simulink library "HyEQ_Library_R2012a"  (R2017a)
settings: Solver=ode45  StartTime=0.0  StopTime=T  MaxStep=MaxStep  RelTol=RelTol  EnableMultiTasking=on
undefined symbols (not defined in the file): C, D, f, g, J, maxU, maxX, minU, rule, T, Tnmax, Tnmin, x0, x0ADC, x0NET
libraries: simulink x24
(part 1 of 3)
settings Model: Creator=pablonanez  LastModifiedBy=pablonanez
settings DataIOCC: LimitDataPoints=on  SaveFormat=Array  SignalLoggingSaveFormat=ModelDataLogs
settings OptimizationCC: ExpressionDepthLimit=2147483647  LifeSpan=inf
settings DebuggingCC: UnderspecifiedInitializationDetection=Classic  MergeDetectMultiDrivingBlocksExec=none  SolverPrmCheckMsg=warning  FcnCallInpInsideContextMsg=warning  StateNameClashWarn=warning  SFUnexpectedBacktrackingDiag=warning  SFNoUnconditionalDefaultTransitionDiag=warning  SFExecutionAtInitializationDiag=none
settings HardwareCC: ProdBitPerPointer=32  ProdBitPerSizeT=32  ProdBitPerPtrDiffT=32  ProdLargestAtomicFloat=None  ProdIntDivRoundTo=Undefined  ProdEndianess=Unspecified  ProdWordSize=32  ProdHWDeviceType=32-bit Generic
settings ModelReferenceCC: PropagateSignalLabelsOutOfModel=off
settings GRTTargetCC: TargetLangStandard=C89/C90 (ANSI)  GeneratePreprocessorConditionals=Disable all  CombineOutputUpdateFcns=off  GRTInterface=on
settings ConfigComp: CovMetricSettings=dw  CovHtmlReporting=on  CovSaveCumulativeToWorkspaceVar=on  CovSaveSingleToWorkspaceVar=on  CovExternalEMLEnable=off

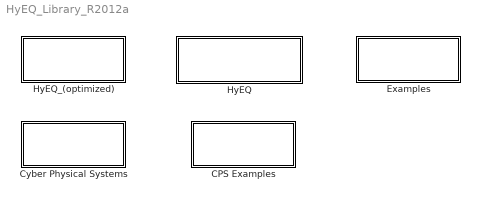
== system HyEQ_Library_R2012a ==
  CPS Examples : Subsystem  LoadFcn=set_param(gcb,'LinkStatus','none')
      settings: CopyFcn=set_param(gcb,'LinkStatus','none')
      mask Display: disp('CPS\n Examples')
  Cyber Physical Systems : Subsystem  LoadFcn=set_param(gcb,'LinkStatus','none')
      settings: CopyFcn=set_param(gcb,'LinkStatus','none')
      mask Display: disp('CPS')
  Examples : Subsystem  LoadFcn=set_param(gcb,'LinkStatus','none')
      settings: CopyFcn=set_param(gcb,'LinkStatus','none')
      mask Display: disp('HyEQ\n Examples')
  HyEQ : Subsystem  LoadFcn=set_param(gcb,'LinkStatus','none')
      settings: CopyFcn=set_param(gcb,'LinkStatus','none')
      mask Display:
      | color('white')
      | 
      | disp('HyEQ \n (No C compiler required)')
  HyEQ_(optimized) : Subsystem  LoadFcn=set_param(gcb,'LinkStatus','none')
      settings: CopyFcn=set_param(gcb,'LinkStatus','none')
      mask Display: disp('HyEQ \n (optimized)')

== system HyEQ_Library_R2012a/CPS Examples ==
  ADC Example 1 : Subsystem  LoadFcn=set_param(gcb,'LinkStatus','none')  mask(Help for the bouncing ball example){}
      mask help: Example: Bouncing ball
      settings: CopyFcn=set_param(gcb,'LinkStatus','none')  OpenFcn=open_system('ADC_example1','force')
      mask Display: disp('ADC example 1')
  ADC Example 2 : Subsystem  LoadFcn=set_param(gcb,'LinkStatus','none')  mask(Help for the bouncing ball example){}
      mask help: Example: Bouncing ball
      settings: CopyFcn=set_param(gcb,'LinkStatus','none')  OpenFcn=open_system('ADC_example2','force')
      mask Display: disp('ADC example 2')
  Continuous Plant : Subsystem  LoadFcn=set_param(gcb,'LinkStatus','none')  mask(Help for the bouncing ball example){}
      mask help: Example: Bouncing ball
      settings: CopyFcn=set_param(gcb,'LinkStatus','none')  OpenFcn=open_system('ContinuousPlant_example','force')
      mask Display: disp('Continuous plant example')
  Finite State Machine Example : Subsystem  LoadFcn=set_param(gcb,'LinkStatus','none')  mask(Help for the bouncing ball example){}
      mask help: Example: Bouncing ball
      settings: CopyFcn=set_param(gcb,'LinkStatus','none')  OpenFcn=open_system('FSM_example','force')
      mask Display: disp('FSM example')
  Networks : Subsystem  LoadFcn=set_param(gcb,'LinkStatus','none')  mask(Help for the bouncing ball example){}
      mask help: Example: Bouncing ball
      settings: CopyFcn=set_param(gcb,'LinkStatus','none')  OpenFcn=open_system('Network_example','force')
      mask Display: disp('Network example')
  Zero Order Hold Example : Subsystem  LoadFcn=set_param(gcb,'LinkStatus','none')  mask(Help for the bouncing ball example){}
      mask help: Example: Bouncing ball
      settings: CopyFcn=set_param(gcb,'LinkStatus','none')  OpenFcn=open_system('ZOH_example','force')
      mask Display: disp('ZOH example')

== system HyEQ_Library_R2012a/Cyber Physical Systems ==
  ADC : Subsystem  LoadFcn=set_param(gcb,'LinkStatus','none')
      settings: CopyFcn=|
      | set_param(gcb,'LinkStatus','none'),
      | set_param(gcs, 'MaxStep', 'MaxStep', 'RelTol', 'RelTol','Stop time', 'T')
      mask Display:
      | image(imread('ADC.jpg'))
      | %plot([5 20 20 5 5],[5 5 20 20 5])
      | %text(8,13,'HyEq_mdl')
      | port_label('output', 1, 'x')
      | port_label('output', 2, 't')
      | port_label('output', 3, 'j')
      | port_label('output', 4, 'x-(int)')
      | port_label('input', 1, 'u')
  FSM : Subsystem  LoadFcn=set_param(gcb,'LinkStatus','none')
      settings: CopyFcn=|
      | set_param(gcb,'LinkStatus','none'),
      | set_param(gcs, 'MaxStep', 'MaxStep', 'RelTol', 'RelTol','Stop time', 'T')
      mask Display:
      | image(imread('FSM.jpg'))
      | %plot([5 20 20 5 5],[5 5 20 20 5])
      | %text(8,13,'HyEq_mdl')
      | port_label('output', 1, 'x')
      | port_label('output', 2, 't')
      | port_label('output', 3, 'j')
      | port_label('output', 4, 'x-(int)')
      | port_label('input', 1, 'u')
  HSu : Subsystem  LoadFcn=set_param(gcb,'LinkStatus','none')
      settings: CopyFcn=|
      | set_param(gcb,'LinkStatus','none'),
      | set_param(gcs, 'MaxStep', 'MaxStep', 'RelTol', 'RelTol','Stop time', 'T')
      mask Display:
      | image(imread('Cplant.jpg'))
      | %plot([5 20 20 5 5],[5 5 20 20 5])
      | %text(8,13,'HyEq_mdl')
      | port_label('output', 1, 'x')
      | port_label('output', 2, 't')
      | port_label('output', 3, 'j')
      | port_label('output', 4, 'x-(int)')
      | port_label('input', 1, 'u')
  ZOH : Subsystem  LoadFcn=set_param(gcb,'LinkStatus','none')
      settings: CopyFcn=|
      | set_param(gcb,'LinkStatus','none'),
      | set_param(gcs, 'MaxStep', 'MaxStep', 'RelTol', 'RelTol','Stop time', 'T')
      mask Display:
      | image(imread('ZOH.jpg'))
      | %plot([5 20 20 5 5],[5 5 20 20 5])
      | %text(8,13,'HyEq_mdl')
      | port_label('output', 1, 'x')
      | port_label('output', 2, 't')
      | port_label('output', 3, 'j')
      | port_label('output', 4, 'x-(int)')
      | port_label('input', 1, 'u')
  network : Subsystem  LoadFcn=set_param(gcb,'LinkStatus','none')
      settings: CopyFcn=|
      | set_param(gcb,'LinkStatus','none'),
      | set_param(gcs, 'MaxStep', 'MaxStep', 'RelTol', 'RelTol','Stop time', 'T')
      mask Display:
      | image(imread('net.jpg'))
      | %plot([5 20 20 5 5],[5 5 20 20 5])
      | %text(8,13,'HyEq_mdl')
      | port_label('output', 1, 'x')
      | port_label('output', 2, 't')
      | port_label('output', 3, 'j')
      | port_label('output', 4, 'x-(int)')
      | port_label('input', 1, 'u')

== system HyEQ_Library_R2012a/Examples ==
  Ex 1.2a Bouncing ball example : Subsystem  LoadFcn=set_param(gcb,'LinkStatus','none')  mask(Help for the bouncing ball example){}
      mask help: Example: Bouncing ball
      settings: CopyFcn=set_param(gcb,'LinkStatus','none')  OpenFcn=open_system('Example_1_2a','force')
      mask Display: disp('Ex 1.2a Bouncing ball \n (external functions)')
  Ex 1.3 Bouncing ball with input : Subsystem  LoadFcn=set_param(gcb,'LinkStatus','none')  mask(Help for the bouncing ball example){}
      mask help: Example: Bouncing ball
      settings: CopyFcn=set_param(gcb,'LinkStatus','none')  OpenFcn=open_system('Example1_3','force')
      mask Display: disp('Ex 1.3 Bouncing ball \n (with input)')
  Ex 1.4 Bouncing ball with operator blocks : Subsystem  LoadFcn=set_param(gcb,'LinkStatus','none')  mask(Help for the bouncing ball example){}
      mask help: Example: Bouncing ball
      settings: CopyFcn=set_param(gcb,'LinkStatus','none')  OpenFcn=open_system('Example1_4','force')
      mask Display: disp('Ex 1.4 Bouncing ball \n (operator blocks)')
  Ex 1.5 Vehicle on Path with Boundaries : Subsystem  LoadFcn=set_param(gcb,'LinkStatus','none')  mask(Help for the bouncing ball example){}
      mask help: Example: Bouncing ball
      settings: CopyFcn=set_param(gcb,'LinkStatus','none')  OpenFcn=open_system('Example1_5','force')
      mask Display: disp('Ex 1.5 Vehicle on Path')
  Ex 1.6 Bouncing Ball and Plataform : Subsystem  LoadFcn=set_param(gcb,'LinkStatus','none')  mask(Help for the bouncing ball example){}
      mask help: Example: Bouncing ball
      settings: CopyFcn=set_param(gcb,'LinkStatus','none')  OpenFcn=open_system('Example1_6','force')
      mask Display: disp('Ex 1.6 Bouncing Ball \n and Moving Platform')
  Ex 1.7 Synchronization of Fireflies : Subsystem  LoadFcn=set_param(gcb,'LinkStatus','none')  mask(Help for the bouncing ball example){}
      mask help: Example: Bouncing ball
      settings: CopyFcn=set_param(gcb,'LinkStatus','none')  OpenFcn=open_system('Example1_7','force')
      mask Display: disp('Ex 1.7 Fireflies')
  Ex 1.8 a Simple Example : Subsystem  LoadFcn=set_param(gcb,'LinkStatus','none')  mask(Help for a simple mathematical example){}
      mask help: Example: a simple mathematical example
      settings: CopyFcn=set_param(gcb,'LinkStatus','none')  OpenFcn=open_system('Ex_1_8_Subblocks','force')
      mask Display: disp('Ex 1.8 a Simple \n Example')

== system HyEQ_Library_R2012a/HyEQ ==
  HS : Subsystem  LoadFcn=set_param(gcb,'LinkStatus','none')
      settings: CopyFcn=|
      | set_param(gcb,'LinkStatus','none'),
      | set_param(gcs, 'MaxStep', 'MaxStep', 'RelTol', 'RelTol')
      mask Display:
      | image(imread('Hcalneg.jpg'))
      | %plot([5 20 20 5 5],[5 5 20 20 5])
      | %text(8,13,'HyEq_mdl')
      | color('white')
      | port_label('output', 1, 'x')
      | port_label('output', 2, 't')
      | port_label('output', 3, 'j')
  Initialize variables : Subsystem  Priority=-10  mask(Initialization file load){}
      mask help: Select the initialization script
      settings: OpenFcn=|
      | try
      |      clearvars -except inifile pathfile_in pathfile_pos posfile
      |      cd(pathfile_in);
      |      eval(inifile);
      | catch
      |      [inifile,pathfile_in] = getInitializationfile;
      |      cd(pathfile_in);
      |      inifile = strrep(inifile,'.m','');
      |      eval(inifile);
      | end
      mask Display: disp('Double Click\n to Initialize')
  More info : Subsystem  mask(Help for HyEQ blocks){}
      mask help: How to use the HyEQ simulink blocks
      settings: OpenFcn=|
      | try
      |      open_system('HyEQ_No_C_Compiler','force')       catch
      | end
      mask Display: disp('Help')
  Plot Solutions : Subsystem  mask(Postprocesing file load){}
      mask help: Select the postprocesing script
      settings: OpenFcn=|
      | try
      |      cd(pathfile_pos);
      |      eval(posfile);
      | catch
      |      [posfile,pathfile_pos] = getInitializationfile;
      |      cd(pathfile_pos);
      |      posfile = strrep(posfile,'.m','');
      |      eval(posfile);
      | end
      mask Display: disp('Double Click to\n Plot Solutions')

== system HyEQ_Library_R2012a/HyEQ_(optimized) ==
  HS : Subsystem  LoadFcn=set_param(gcb,'LinkStatus','none')
      settings: CopyFcn=|
      | set_param(gcb,'LinkStatus','none'),
      | set_param(gcs, 'MaxStep', 'MaxStep', 'RelTol', 'RelTol','Stop time', 'T')
      mask Display:
      | image(imread('Hcal.jpg'))
      | %plot([5 20 20 5 5],[5 5 20 20 5])
      | %text(8,13,'HyEq_mdl')
      | port_label('output', 1, 'x')
      | port_label('output', 2, 't')
      | port_label('output', 3, 'j')
  HSu : Subsystem  LoadFcn=set_param(gcb,'LinkStatus','none')
      settings: CopyFcn=|
      | set_param(gcb,'LinkStatus','none'),
      | set_param(gcs, 'MaxStep', 'MaxStep', 'RelTol', 'RelTol','Stop time', 'T')
      mask Display:
      | image(imread('Hcal.jpg'))
      | %plot([5 20 20 5 5],[5 5 20 20 5])
      | %text(8,13,'HyEq_mdl')
      | port_label('output', 1, 'x')
      | port_label('output', 2, 't')
      | port_label('output', 3, 'j')
      | port_label('output', 4, 'x-(int)')
      | port_label('input', 1, 'u')
  Initialize variables : Subsystem  Priority=-10  mask(Initialization file load){}
      mask help: Select the initialization script
      settings: OpenFcn=|
      | try
      |      clearvars -except inifile pathfile_in pathfile_pos posfile
      |      cd(pathfile_in);
      |      eval(inifile);
      | catch
      |      [inifile,pathfile_in] = getInitializationfile;
      |      cd(pathfile_in);
      |      inifile = strrep(inifile,'.m','');
      |      eval(inifile);
      | end
      mask Display: disp('Double Click\n to Initialize')
  More info : Subsystem  mask(Help for HyEQ blocks){}
      mask help: How to use the HyEQ simulink blocks
      settings: OpenFcn=|
      | try
      |      open_system('HyEQ_Optimized','force')
      | catch
      | end
      mask Display: disp('Help')
  Plot Solutions : Subsystem  mask(Postprocesing file load){}
      mask help: Select the postprocesing script
      settings: OpenFcn=|
      | try
      |      cd(pathfile_pos);
      |      eval(posfile);
      | catch
      |      [posfile,pathfile_pos] = getInitializationfile;
      |      cd(pathfile_pos);
      |      posfile = strrep(posfile,'.m','');
      |      eval(posfile);
      | end
      mask Display: disp('Double Click to\n Plot Solutions')

== system HyEQ_Library_R2012a/CPS Examples/ADC Example 1 ==
  Gain : Gain

== system HyEQ_Library_R2012a/CPS Examples/ADC Example 2 ==
  Gain : Gain

== system HyEQ_Library_R2012a/CPS Examples/Continuous Plant ==
  Gain : Gain

== system HyEQ_Library_R2012a/CPS Examples/Finite State Machine Example ==
  Gain : Gain

== system HyEQ_Library_R2012a/CPS Examples/Networks ==
  Gain : Gain

== system HyEQ_Library_R2012a/CPS Examples/Zero Order Hold Example ==
  Gain : Gain

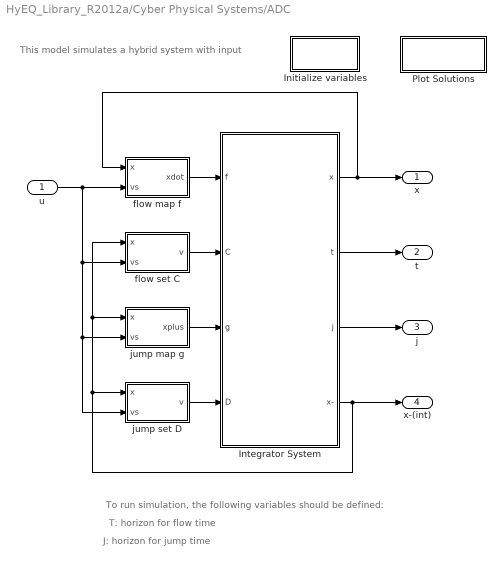
== system HyEQ_Library_R2012a/Cyber Physical Systems/ADC ==
  note: This model simulates a hybrid system with input
  note: To run simulation, the following variables should be defined:
  note: T: horizon for flow time
  note: J: horizon for jump time
  u : Inport
  Initialize variables : Subsystem  Priority=-10
      settings: OpenFcn=|
      | try
      |      clearvars -except inifile pathfile_in pathfile_pos posfile
      |      cd(pathfile_in);
      |      eval(inifile);
      | catch
      |      [inifile,pathfile_in] = getInitializationfile;
      |      cd(pathfile_in);
      |      inifile = strrep(inifile,'.m','');
      |      eval(inifile);
      | end
      mask Display: disp('Double Click\n to Initialize')
  Integrator System : Subsystem  Priority=2  mask(Hybrid Integrator){T=T, J=J, x0=x0ADC}
      mask prompts: T "Flow Horizon"; J "Jump Horizon"; x0 "Initial Condition"
      mask help:
      | This block integrates the state of the hybrid system defined by the flow map f (first input), the flow set C (second input), the jump map g (third input) and the jump set D (fourth input).
      | Starting from the initial condition x0 (last mask parameter), the system's state x evolves continuously within the set C, according to f(x,u), but is also subject to jumps within D, according to g(x,u).
      | The block also stops the simulation when the time t is greater than the flow horizon T (first mask parameter), or when the number of jumps j is greater than the jump horizon J (second mask parameter).
      | The outputs of the blocks are respectively x(t), t, j, x(t-).
      mask Help:
      | This block integrates the state of the hybrid system defined by the flow map f (first input), the flow set C (second input), the jump map g (third input) and the jump set D (fourth input).
      | <br>
      | Starting from the initial condition x0 (last mask parameter), the system's state x evolves continuously within the set C, according to f(x,u), but is also subject to jumps within D, according to g(x,u).
      | <br>
      | The block also stops the simulation when the time t is greater than the flow horizon T (first mask parameter), or when the number of jumps j is greater than the jump horizon J (second mask parameter).
      | <br>
      | The outputs of the blocks are respectively x(t), t, j, x(t-).
      | <br>
      | You can right click on the block and "Look under mask" to see what's inside the block.
      | Finally, refer to the manual (HybridSimulator_vXX.pdf) for more detailed information on how this hybrid simulator works.
  Plot Solutions : Subsystem
      settings: OpenFcn=|
      | try
      |      cd(pathfile_pos);
      |      eval(posfile);
      | catch
      |      [posfile,pathfile_pos] = getInitializationfile;
      |      cd(pathfile_pos);
      |      posfile = strrep(posfile,'.m','');
      |      eval(posfile);
      | end
      mask Display: disp('Double Click to\n Plot Solutions')
  flow map f : MATLAB Function  TreatAsAtomicUnit=on
  flow set C : MATLAB Function  TreatAsAtomicUnit=on
  jump map g : MATLAB Function  Priority=2  TreatAsAtomicUnit=on
  jump set D : MATLAB Function  TreatAsAtomicUnit=on
  x : Outport
  t : Outport  Port=2
  j : Outport  Port=3
  x-(int) : Outport  Port=4
  wires:
  flow map f/1(xdot) -> Integrator System/1(f)
  Integrator System/4(x-) -> jump map g/1(x), flow set C/1(x), jump set D/1(x), x-(int)/1
  Integrator System/1(x) -> flow map f/1(x), x/1
  flow set C/1(v) -> Integrator System/2(C)
  Integrator System/2(t) -> t/1
  Integrator System/3(j) -> j/1
  u/1 -> flow map f/2(vs), flow set C/2(vs), jump map g/2(vs), jump set D/2(vs)
  jump set D/1(v) -> Integrator System/4(D)
  jump map g/1(xplus) -> Integrator System/3(g)

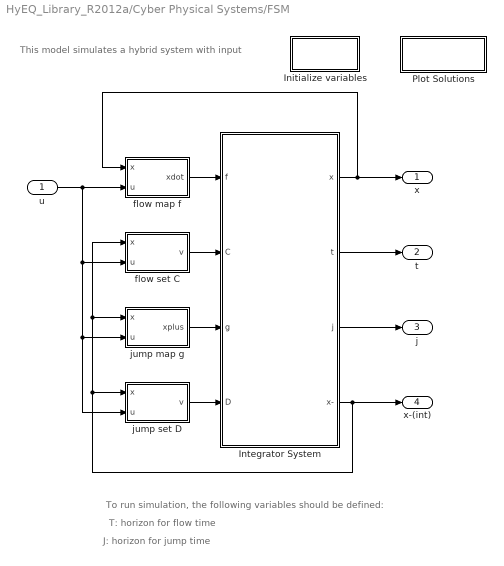
== system HyEQ_Library_R2012a/Cyber Physical Systems/FSM ==
  note: This model simulates a hybrid system with input
  note: To run simulation, the following variables should be defined:
  note: T: horizon for flow time
  note: J: horizon for jump time
  u : Inport
  Initialize variables : Subsystem  Priority=-10
      settings: OpenFcn=|
      | try
      |      clearvars -except inifile pathfile_in pathfile_pos posfile
      |      cd(pathfile_in);
      |      eval(inifile);
      | catch
      |      [inifile,pathfile_in] = getInitializationfile;
      |      cd(pathfile_in);
      |      inifile = strrep(inifile,'.m','');
      |      eval(inifile);
      | end
      mask Display: disp('Double Click\n to Initialize')
  Integrator System : Subsystem  Priority=2  mask(Hybrid Integrator){T=T, J=J, x0=x0}
      mask prompts: T "Flow Horizon"; J "Jump Horizon"; x0 "Initial Condition"
      mask help:
      | This block integrates the state of the hybrid system defined by the flow map f (first input), the flow set C (second input), the jump map g (third input) and the jump set D (fourth input).
      | Starting from the initial condition x0 (last mask parameter), the system's state x evolves continuously within the set C, according to f(x,u), but is also subject to jumps within D, according to g(x,u).
      | The block also stops the simulation when the time t is greater than the flow horizon T (first mask parameter), or when the number of jumps j is greater than the jump horizon J (second mask parameter).
      | The outputs of the blocks are respectively x(t), t, j, x(t-).
      mask Help:
      | This block integrates the state of the hybrid system defined by the flow map f (first input), the flow set C (second input), the jump map g (third input) and the jump set D (fourth input).
      | <br>
      | Starting from the initial condition x0 (last mask parameter), the system's state x evolves continuously within the set C, according to f(x,u), but is also subject to jumps within D, according to g(x,u).
      | <br>
      | The block also stops the simulation when the time t is greater than the flow horizon T (first mask parameter), or when the number of jumps j is greater than the jump horizon J (second mask parameter).
      | <br>
      | The outputs of the blocks are respectively x(t), t, j, x(t-).
      | <br>
      | You can right click on the block and "Look under mask" to see what's inside the block.
      | Finally, refer to the manual (HybridSimulator_vXX.pdf) for more detailed information on how this hybrid simulator works.
  Plot Solutions : Subsystem
      settings: OpenFcn=|
      | try
      |      cd(pathfile_pos);
      |      eval(posfile);
      | catch
      |      [posfile,pathfile_pos] = getInitializationfile;
      |      cd(pathfile_pos);
      |      posfile = strrep(posfile,'.m','');
      |      eval(posfile);
      | end
      mask Display: disp('Double Click to\n Plot Solutions')
  flow map f : MATLAB Function  TreatAsAtomicUnit=on
  flow set C : MATLAB Function  TreatAsAtomicUnit=on
  jump map g : MATLAB Function  Priority=2  TreatAsAtomicUnit=on
  jump set D : MATLAB Function  TreatAsAtomicUnit=on
  x : Outport
  t : Outport  Port=2
  j : Outport  Port=3
  x-(int) : Outport  Port=4
  wires:
  flow map f/1(xdot) -> Integrator System/1(f)
  Integrator System/4(x-) -> jump map g/1(x), flow set C/1(x), jump set D/1(x), x-(int)/1
  Integrator System/1(x) -> flow map f/1(x), x/1
  flow set C/1(v) -> Integrator System/2(C)
  Integrator System/2(t) -> t/1
  Integrator System/3(j) -> j/1
  u/1 -> flow map f/2(u), flow set C/2(u), jump map g/2(u), jump set D/2(u)
  jump set D/1(v) -> Integrator System/4(D)
  jump map g/1(xplus) -> Integrator System/3(g)

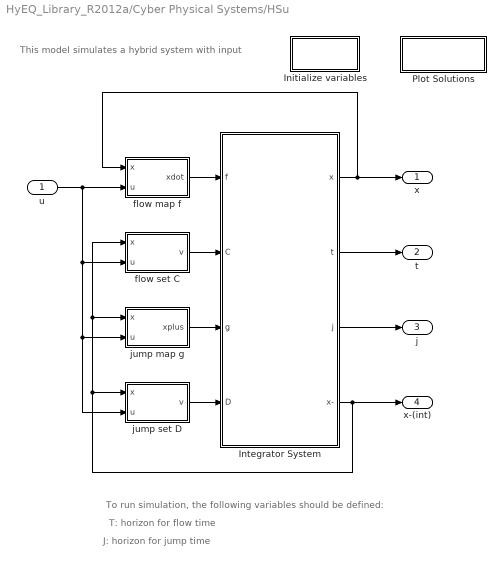
== system HyEQ_Library_R2012a/Cyber Physical Systems/HSu ==
  note: This model simulates a hybrid system with input
  note: To run simulation, the following variables should be defined:
  note: T: horizon for flow time
  note: J: horizon for jump time
  u : Inport
  Initialize variables : Subsystem  Priority=-10
      settings: OpenFcn=|
      | try
      |      clearvars -except inifile pathfile_in pathfile_pos posfile
      |      cd(pathfile_in);
      |      eval(inifile);
      | catch
      |      [inifile,pathfile_in] = getInitializationfile;
      |      cd(pathfile_in);
      |      inifile = strrep(inifile,'.m','');
      |      eval(inifile);
      | end
      mask Display: disp('Double Click\n to Initialize')
  Integrator System : Subsystem  Priority=2  mask(Hybrid Integrator){T=T, J=J, x0=x0}
      mask prompts: T "Flow Horizon"; J "Jump Horizon"; x0 "Initial Condition"
      mask help:
      | This block integrates the state of the hybrid system defined by the flow map f (first input), the flow set C (second input), the jump map g (third input) and the jump set D (fourth input).
      | Starting from the initial condition x0 (last mask parameter), the system's state x evolves continuously within the set C, according to f(x,u), but is also subject to jumps within D, according to g(x,u).
      | The block also stops the simulation when the time t is greater than the flow horizon T (first mask parameter), or when the number of jumps j is greater than the jump horizon J (second mask parameter).
      | The outputs of the blocks are respectively x(t), t, j, x(t-).
      mask Help:
      | This block integrates the state of the hybrid system defined by the flow map f (first input), the flow set C (second input), the jump map g (third input) and the jump set D (fourth input).
      | <br>
      | Starting from the initial condition x0 (last mask parameter), the system's state x evolves continuously within the set C, according to f(x,u), but is also subject to jumps within D, according to g(x,u).
      | <br>
      | The block also stops the simulation when the time t is greater than the flow horizon T (first mask parameter), or when the number of jumps j is greater than the jump horizon J (second mask parameter).
      | <br>
      | The outputs of the blocks are respectively x(t), t, j, x(t-).
      | <br>
      | You can right click on the block and "Look under mask" to see what's inside the block.
      | Finally, refer to the manual (HybridSimulator_vXX.pdf) for more detailed information on how this hybrid simulator works.
  Plot Solutions : Subsystem
      settings: OpenFcn=|
      | try
      |      cd(pathfile_pos);
      |      eval(posfile);
      | catch
      |      [posfile,pathfile_pos] = getInitializationfile;
      |      cd(pathfile_pos);
      |      posfile = strrep(posfile,'.m','');
      |      eval(posfile);
      | end
      mask Display: disp('Double Click to\n Plot Solutions')
  flow map f : MATLAB Function  TreatAsAtomicUnit=on
  flow set C : MATLAB Function  TreatAsAtomicUnit=on
  jump map g : MATLAB Function  Priority=2  TreatAsAtomicUnit=on
  jump set D : MATLAB Function  TreatAsAtomicUnit=on
  x : Outport
  t : Outport  Port=2
  j : Outport  Port=3
  x-(int) : Outport  Port=4
  wires:
  flow map f/1(xdot) -> Integrator System/1(f)
  Integrator System/4(x-) -> jump map g/1(x), flow set C/1(x), jump set D/1(x), x-(int)/1
  Integrator System/1(x) -> flow map f/1(x), x/1
  flow set C/1(v) -> Integrator System/2(C)
  Integrator System/2(t) -> t/1
  Integrator System/3(j) -> j/1
  u/1 -> flow map f/2(u), flow set C/2(u), jump map g/2(u), jump set D/2(u)
  jump set D/1(v) -> Integrator System/4(D)
  jump map g/1(xplus) -> Integrator System/3(g)

== system HyEQ_Library_R2012a/Cyber Physical Systems/ZOH ==
  note: This model simulates a hybrid system with input
  note: To run simulation, the following variables should be defined:
  note: T: horizon for flow time
  note: J: horizon for jump time
  u : Inport
  Initialize variables : Subsystem  Priority=-10
      settings: OpenFcn=|
      | try
      |      clearvars -except inifile pathfile_in pathfile_pos posfile
      |      cd(pathfile_in);
      |      eval(inifile);
      | catch
      |      [inifile,pathfile_in] = getInitializationfile;
      |      cd(pathfile_in);
      |      inifile = strrep(inifile,'.m','');
      |      eval(inifile);
      | end
      mask Display: disp('Double Click\n to Initialize')
  Integrator System : Subsystem  Priority=2  mask(Hybrid Integrator){T=T, J=J, x0=x0ADC}
      mask prompts: T "Flow Horizon"; J "Jump Horizon"; x0 "Initial Condition"
      mask help:
      | This block integrates the state of the hybrid system defined by the flow map f (first input), the flow set C (second input), the jump map g (third input) and the jump set D (fourth input).
      | Starting from the initial condition x0 (last mask parameter), the system's state x evolves continuously within the set C, according to f(x,u), but is also subject to jumps within D, according to g(x,u).
      | The block also stops the simulation when the time t is greater than the flow horizon T (first mask parameter), or when the number of jumps j is greater than the jump horizon J (second mask parameter).
      | The outputs of the blocks are respectively x(t), t, j, x(t-).
      mask Help:
      | This block integrates the state of the hybrid system defined by the flow map f (first input), the flow set C (second input), the jump map g (third input) and the jump set D (fourth input).
      | <br>
      | Starting from the initial condition x0 (last mask parameter), the system's state x evolves continuously within the set C, according to f(x,u), but is also subject to jumps within D, according to g(x,u).
      | <br>
      | The block also stops the simulation when the time t is greater than the flow horizon T (first mask parameter), or when the number of jumps j is greater than the jump horizon J (second mask parameter).
      | <br>
      | The outputs of the blocks are respectively x(t), t, j, x(t-).
      | <br>
      | You can right click on the block and "Look under mask" to see what's inside the block.
      | Finally, refer to the manual (HybridSimulator_vXX.pdf) for more detailed information on how this hybrid simulator works.
  Plot Solutions : Subsystem
      settings: OpenFcn=|
      | try
      |      cd(pathfile_pos);
      |      eval(posfile);
      | catch
      |      [posfile,pathfile_pos] = getInitializationfile;
      |      cd(pathfile_pos);
      |      posfile = strrep(posfile,'.m','');
      |      eval(posfile);
      | end
      mask Display: disp('Double Click to\n Plot Solutions')
  flow map f : MATLAB Function  TreatAsAtomicUnit=on
  flow set C : MATLAB Function  TreatAsAtomicUnit=on
  jump map g : MATLAB Function  Priority=2  TreatAsAtomicUnit=on
  jump set D : MATLAB Function  TreatAsAtomicUnit=on
  x : Outport
  t : Outport  Port=2
  j : Outport  Port=3
  x-(int) : Outport  Port=4
  wires:
  flow map f/1(xdot) -> Integrator System/1(f)
  Integrator System/4(x-) -> jump map g/1(x), flow set C/1(x), jump set D/1(x), x-(int)/1
  Integrator System/1(x) -> flow map f/1(x), x/1
  flow set C/1(v) -> Integrator System/2(C)
  Integrator System/2(t) -> t/1
  Integrator System/3(j) -> j/1
  u/1 -> flow map f/2(vs), flow set C/2(vs), jump map g/2(vs), jump set D/2(vs)
  jump set D/1(v) -> Integrator System/4(D)
  jump map g/1(xplus) -> Integrator System/3(g)

== system HyEQ_Library_R2012a/Cyber Physical Systems/network ==
  note: This model simulates a hybrid system with input
  note: To run simulation, the following variables should be defined:
  note: T: horizon for flow time
  note: J: horizon for jump time
  u : Inport
  Initialize variables : Subsystem  Priority=-10
      settings: OpenFcn=|
      | try
      |      clearvars -except inifile pathfile_in pathfile_pos posfile
      |      cd(pathfile_in);
      |      eval(inifile);
      | catch
      |      [inifile,pathfile_in] = getInitializationfile;
      |      cd(pathfile_in);
      |      inifile = strrep(inifile,'.m','');
      |      eval(inifile);
      | end
      mask Display: disp('Double Click\n to Initialize')
  Integrator System : Subsystem  Priority=2  mask(Hybrid Integrator){T=T, J=J, x0=x0NET}
      mask prompts: T "Flow Horizon"; J "Jump Horizon"; x0 "Initial Condition"
      mask help:
      | This block integrates the state of the hybrid system defined by the flow map f (first input), the flow set C (second input), the jump map g (third input) and the jump set D (fourth input).
      | Starting from the initial condition x0 (last mask parameter), the system's state x evolves continuously within the set C, according to f(x,u), but is also subject to jumps within D, according to g(x,u).
      | The block also stops the simulation when the time t is greater than the flow horizon T (first mask parameter), or when the number of jumps j is greater than the jump horizon J (second mask parameter).
      | The outputs of the blocks are respectively x(t), t, j, x(t-).
      mask Help:
      | This block integrates the state of the hybrid system defined by the flow map f (first input), the flow set C (second input), the jump map g (third input) and the jump set D (fourth input).
      | <br>
      | Starting from the initial condition x0 (last mask parameter), the system's state x evolves continuously within the set C, according to f(x,u), but is also subject to jumps within D, according to g(x,u).
      | <br>
      | The block also stops the simulation when the time t is greater than the flow horizon T (first mask parameter), or when the number of jumps j is greater than the jump horizon J (second mask parameter).
      | <br>
      | The outputs of the blocks are respectively x(t), t, j, x(t-).
      | <br>
      | You can right click on the block and "Look under mask" to see what's inside the block.
      | Finally, refer to the manual (HybridSimulator_vXX.pdf) for more detailed information on how this hybrid simulator works.
  Plot Solutions : Subsystem
      settings: OpenFcn=|
      | try
      |      cd(pathfile_pos);
      |      eval(posfile);
      | catch
      |      [posfile,pathfile_pos] = getInitializationfile;
      |      cd(pathfile_pos);
      |      posfile = strrep(posfile,'.m','');
      |      eval(posfile);
      | end
      mask Display: disp('Double Click to\n Plot Solutions')
  flow map f : MATLAB Function  TreatAsAtomicUnit=on
  flow set C : MATLAB Function  TreatAsAtomicUnit=on
  jump map g : MATLAB Function  Priority=2  TreatAsAtomicUnit=on
  jump set D : MATLAB Function  TreatAsAtomicUnit=on
  x : Outport
  t : Outport  Port=2
  j : Outport  Port=3
  x-(int) : Outport  Port=4
  wires:
  flow map f/1(xdot) -> Integrator System/1(f)
  Integrator System/4(x-) -> jump map g/1(x), flow set C/1(x), jump set D/1(x), x-(int)/1
  Integrator System/1(x) -> flow map f/1(x), x/1
  flow set C/1(v) -> Integrator System/2(C)
  Integrator System/2(t) -> t/1
  Integrator System/3(j) -> j/1
  u/1 -> flow map f/2(vs), flow set C/2(vs), jump map g/2(vs), jump set D/2(vs)
  jump set D/1(v) -> Integrator System/4(D)
  jump map g/1(xplus) -> Integrator System/3(g)

== system HyEQ_Library_R2012a/Examples/Ex 1.2a Bouncing ball example ==
  Gain : Gain

== system HyEQ_Library_R2012a/Examples/Ex 1.3 Bouncing ball with input ==
  Gain : Gain

== system HyEQ_Library_R2012a/Examples/Ex 1.4 Bouncing ball with operator blocks ==
  Gain : Gain

== system HyEQ_Library_R2012a/Examples/Ex 1.5 Vehicle on Path with Boundaries ==
  Gain : Gain

== system HyEQ_Library_R2012a/Examples/Ex 1.6 Bouncing Ball and Plataform ==
  Gain : Gain

== system HyEQ_Library_R2012a/Examples/Ex 1.7 Synchronization of Fireflies ==
  Gain : Gain

== system HyEQ_Library_R2012a/Examples/Ex 1.8 a Simple Example ==
  Gain : Gain

== system HyEQ_Library_R2012a/HyEQ/HS ==
  note: This model simulates a hybrid system
  Initialize variables : Subsystem  Priority=-10
      settings: OpenFcn=|
      | try
      |      clearvars -except inifile pathfile_in pathfile_pos posfile
      |      cd(pathfile_in);
      |      eval(inifile);
      | catch
      |      [inifile,pathfile_in] = getInitializationfile;
      |      cd(pathfile_in);
      |      inifile = strrep(inifile,'.m','');
      |      eval(inifile);
      | end
      mask Display: disp('Double Click\n to Initialize')
  Integrator System : Subsystem  Priority=2  mask(Hybrid Integrator){T=T, J=J, x0=x0}
      mask prompts: T "Flow Horizon"; J "Jump Horizon"; x0 "Initial Condition"
      mask help:
      | This block integrates the state of the hybrid system defined by the flow map f (first input), the flow set C (second input), the jump map g (third input) and the jump set D (fourth input).
      | Starting from the initial condition x0 (last mask parameter), the system's state x evolves continuously within the set C, according to f(x,u), but is also subject to jumps within D, according to g(x,u).
      | The block also stops the simulation when the time t is greater than the flow horizon T (first mask parameter), or when the number of jumps j is greater than the jump horizon J (second mask parameter).
      | The outputs of the blocks are respectively x(t), t, j, x(t-).
      mask Help:
      | This block integrates the state of the hybrid system defined by the flow map f (first input), the flow set C (second input), the jump map g (third input) and the jump set D (fourth input).
      | <br>
      | Starting from the initial condition x0 (last mask parameter), the system's state x evolves continuously within the set C, according to f(x,u), but is also subject to jumps within D, according to g(x,u).
      | <br>
      | The block also stops the simulation when the time t is greater than the flow horizon T (first mask parameter), or when the number of jumps j is greater than the jump horizon J (second mask parameter).
      | <br>
      | The outputs of the blocks are respectively x(t), t, j, x(t-).
      | <br>
      | You can right click on the block and "Look under mask" to see what's inside the block.
      | Finally, refer to the manual (HybridSimulator_vXX.pdf) for more detailed information on how this hybrid simulator works.
  Plot Solutions : Subsystem
      settings: OpenFcn=|
      | try
      |      cd(pathfile_pos);
      |      eval(posfile);
      | catch
      |      [posfile,pathfile_pos] = getInitializationfile;
      |      cd(pathfile_pos);
      |      posfile = strrep(posfile,'.m','');
      |      eval(posfile);
      | end
      mask Display: disp('Double Click to\n Plot Solutions')
  flow map f : MATLABFcn  MATLABFcn=f(u)
  flow set C : MATLABFcn  MATLABFcn=C(u)
  jump map g : MATLABFcn  MATLABFcn=g(u)
  jump set D : MATLABFcn  MATLABFcn=D(u)
  x : Outport
  t : Outport  Port=2
  j : Outport  Port=3
  wires:
  jump map g/1 -> Integrator System/3(g)
  jump set D/1 -> Integrator System/4(D)
  Integrator System/3(j) -> j/1
  Integrator System/2(t) -> t/1
  flow set C/1 -> Integrator System/2(C)
  Integrator System/1(x) -> flow map f/1, x/1
  Integrator System/4(x-) -> flow set C/1, jump map g/1, jump set D/1
  flow map f/1 -> Integrator System/1(f)

== system HyEQ_Library_R2012a/HyEQ/Initialize variables ==
  Gain : Gain

== system HyEQ_Library_R2012a/HyEQ/More info ==
  Gain : Gain

== system HyEQ_Library_R2012a/HyEQ/Plot Solutions ==
  Gain : Gain

== system HyEQ_Library_R2012a/HyEQ_(optimized)/HS ==
  note: This model simulates a hybrid system with input
  note: To run simulation, the following variables should be defined:
  note: T: horizon for flow time
  note: J: horizon for jump time
  Initialize variables : Subsystem  Priority=-10
      settings: OpenFcn=|
      | try
      |      clearvars -except inifile pathfile_in pathfile_pos posfile
      |      cd(pathfile_in);
      |      eval(inifile);
      | catch
      |      [inifile,pathfile_in] = getInitializationfile;
      |      cd(pathfile_in);
      |      inifile = strrep(inifile,'.m','');
      |      eval(inifile);
      | end
      mask Display: disp('Double Click\n to Initialize')
  Integrator System : Subsystem  Priority=2  mask(Hybrid Integrator){T=T, J=J, x0=x0}
      mask prompts: T "Flow Horizon"; J "Jump Horizon"; x0 "Initial Condition"
      mask help:
      | This block integrates the state of the hybrid system defined by the flow map f (first input), the flow set C (second input), the jump map g (third input) and the jump set D (fourth input).
      | Starting from the initial condition x0 (last mask parameter), the system's state x evolves continuously within the set C, according to f(x,u), but is also subject to jumps within D, according to g(x,u).
      | The block also stops the simulation when the time t is greater than the flow horizon T (first mask parameter), or when the number of jumps j is greater than the jump horizon J (second mask parameter).
      | The outputs of the blocks are respectively x(t), t, j, x(t-).
      mask Help:
      | This block integrates the state of the hybrid system defined by the flow map f (first input), the flow set C (second input), the jump map g (third input) and the jump set D (fourth input).
      | <br>
      | Starting from the initial condition x0 (last mask parameter), the system's state x evolves continuously within the set C, according to f(x,u), but is also subject to jumps within D, according to g(x,u).
      | <br>
      | The block also stops the simulation when the time t is greater than the flow horizon T (first mask parameter), or when the number of jumps j is greater than the jump horizon J (second mask parameter).
      | <br>
      | The outputs of the blocks are respectively x(t), t, j, x(t-).
      | <br>
      | You can right click on the block and "Look under mask" to see what's inside the block.
      | Finally, refer to the manual (HybridSimulator_vXX.pdf) for more detailed information on how this hybrid simulator works.
  Plot Solutions : Subsystem
      settings: OpenFcn=|
      | try
      |      cd(pathfile_pos);
      |      eval(posfile);
      | catch
      |      [posfile,pathfile_pos] = getInitializationfile;
      |      cd(pathfile_pos);
      |      posfile = strrep(posfile,'.m','');
      |      eval(posfile);
      | end
      mask Display: disp('Double Click to\n Plot Solutions')
  flow map f : MATLAB Function  TreatAsAtomicUnit=on
  flow set C : MATLAB Function  TreatAsAtomicUnit=on
  jump map g : MATLAB Function  Priority=2  TreatAsAtomicUnit=on
  jump set D : MATLAB Function  TreatAsAtomicUnit=on
  x : Outport
  t : Outport  Port=2
  j : Outport  Port=3
  wires:
  flow map f/1(xdot) -> Integrator System/1(f)
  Integrator System/4(x-) -> jump map g/1(x), flow set C/1(x), jump set D/1(x)
  Integrator System/1(x) -> flow map f/1(x), x/1
  flow set C/1(v) -> Integrator System/2(C)
  Integrator System/2(t) -> t/1
  Integrator System/3(j) -> j/1
  jump set D/1(v) -> Integrator System/4(D)
  jump map g/1(xplus) -> Integrator System/3(g)

== system HyEQ_Library_R2012a/HyEQ_(optimized)/HSu ==
  note: This model simulates a hybrid system with input
  note: To run simulation, the following variables should be defined:
  note: T: horizon for flow time
  note: J: horizon for jump time
  u : Inport
  Initialize variables : Subsystem  Priority=-10
      settings: OpenFcn=|
      | try
      |      clearvars -except inifile pathfile_in pathfile_pos posfile
      |      cd(pathfile_in);
      |      eval(inifile);
      | catch
      |      [inifile,pathfile_in] = getInitializationfile;
      |      cd(pathfile_in);
      |      inifile = strrep(inifile,'.m','');
      |      eval(inifile);
      | end
      mask Display: disp('Double Click\n to Initialize')
  Integrator System : Subsystem  Priority=2  mask(Hybrid Integrator){T=T, J=J, x0=x0}
      mask prompts: T "Flow Horizon"; J "Jump Horizon"; x0 "Initial Condition"
      mask help:
      | This block integrates the state of the hybrid system defined by the flow map f (first input), the flow set C (second input), the jump map g (third input) and the jump set D (fourth input).
      | Starting from the initial condition x0 (last mask parameter), the system's state x evolves continuously within the set C, according to f(x,u), but is also subject to jumps within D, according to g(x,u).
      | The block also stops the simulation when the time t is greater than the flow horizon T (first mask parameter), or when the number of jumps j is greater than the jump horizon J (second mask parameter).
      | The outputs of the blocks are respectively x(t), t, j, x(t-).
      mask Help:
      | This block integrates the state of the hybrid system defined by the flow map f (first input), the flow set C (second input), the jump map g (third input) and the jump set D (fourth input).
      | <br>
      | Starting from the initial condition x0 (last mask parameter), the system's state x evolves continuously within the set C, according to f(x,u), but is also subject to jumps within D, according to g(x,u).
      | <br>
      | The block also stops the simulation when the time t is greater than the flow horizon T (first mask parameter), or when the number of jumps j is greater than the jump horizon J (second mask parameter).
      | <br>
      | The outputs of the blocks are respectively x(t), t, j, x(t-).
      | <br>
      | You can right click on the block and "Look under mask" to see what's inside the block.
      | Finally, refer to the manual (HybridSimulator_vXX.pdf) for more detailed information on how this hybrid simulator works.
  Plot Solutions : Subsystem
      settings: OpenFcn=|
      | try
      |      cd(pathfile_pos);
      |      eval(posfile);
      | catch
      |      [posfile,pathfile_pos] = getInitializationfile;
      |      cd(pathfile_pos);
      |      posfile = strrep(posfile,'.m','');
      |      eval(posfile);
      | end
      mask Display: disp('Double Click to\n Plot Solutions')
  flow map f : MATLAB Function  TreatAsAtomicUnit=on
  flow set C : MATLAB Function  TreatAsAtomicUnit=on
  jump map g : MATLAB Function  Priority=2  TreatAsAtomicUnit=on
  jump set D : MATLAB Function  TreatAsAtomicUnit=on
  x : Outport
  t : Outport  Port=2
  j : Outport  Port=3
  x-(int) : Outport  Port=4
  wires:
  flow map f/1(xdot) -> Integrator System/1(f)
  Integrator System/4(x-) -> jump map g/1(x), flow set C/1(x), jump set D/1(x), x-(int)/1
  Integrator System/1(x) -> flow map f/1(x), x/1
  flow set C/1(v) -> Integrator System/2(C)
  Integrator System/2(t) -> t/1
  Integrator System/3(j) -> j/1
  u/1 -> flow map f/2(u), flow set C/2(u), jump map g/2(u), jump set D/2(u)
  jump set D/1(v) -> Integrator System/4(D)
  jump map g/1(xplus) -> Integrator System/3(g)

== system HyEQ_Library_R2012a/HyEQ_(optimized)/Initialize variables ==
  Gain : Gain

== system HyEQ_Library_R2012a/HyEQ_(optimized)/More info ==
  Gain : Gain

== system HyEQ_Library_R2012a/HyEQ_(optimized)/Plot Solutions ==
  Gain : Gain

== system HyEQ_Library_R2012a/Cyber Physical Systems/ADC/Initialize variables ==

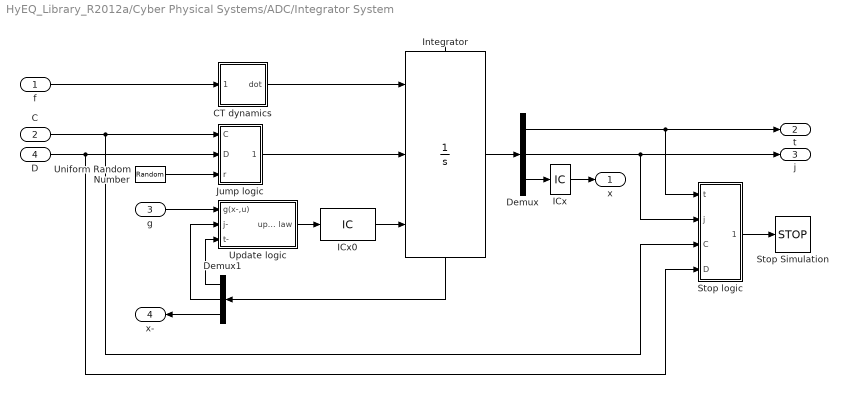
== system HyEQ_Library_R2012a/Cyber Physical Systems/ADC/Integrator System ==
  f : Inport
  C : Inport  Port=2
  g : Inport  Port=3
  D : Inport  Port=4
  CT dynamics : Subsystem
  Demux : Demux  Outputs=[1 1 -1]
  Demux1 : Demux  Outputs=[1 1 -1]
  ICx : InitialCondition  Value=x0
  ICx0 : InitialCondition  Value=[0; 0; x0(:)]
  Integrator : Integrator  ExternalReset=level hold  InitialConditionSource=external  ShowStatePort=on  ZeroCross=off
  Jump logic : Subsystem
  Stop Simulation : Stop
  Stop logic : Subsystem
  Uniform Random Number : UniformRandomNumber  Minimum=0  Seed=abs(floor(100*rand))  SampleTime=0
  Update logic : Subsystem
  x : Outport
  t : Outport  Port=2
  j : Outport  Port=3
  x- : Outport  Port=4
  wires:
  Demux1/2 -> Update logic/2(j-)
  Demux1/1 -> Update logic/3(t-)
  g/1 -> Update logic/1(g(x-,u))
  Uniform Random Number/1 -> Jump logic/3(r)
  Jump logic/1(jump) -> Integrator/2
  Demux1/3 -> x-/1
  f/1 -> CT dynamics/1(f(x,u))
  D/1 -> Jump logic/2(D), Stop logic/4(D)
  C/1 -> Jump logic/1(C), Stop logic/3(C)
  Integrator/1 -> Demux/1
  Stop logic/1(stop) -> Stop Simulation/1
  CT dynamics/1(dot) -> Integrator/1
  Update logic/1(update law) -> ICx0/1
  Demux/1 -> Stop logic/1(t), t/1
  Demux/2 -> Stop logic/2(j), j/1
  Integrator/State -> Demux1/1
  Demux/3 -> ICx/1
  ICx/1 -> x/1
  ICx0/1 -> Integrator/3

== system HyEQ_Library_R2012a/Cyber Physical Systems/ADC/Plot Solutions ==

== system HyEQ_Library_R2012a/Cyber Physical Systems/FSM/Initialize variables ==

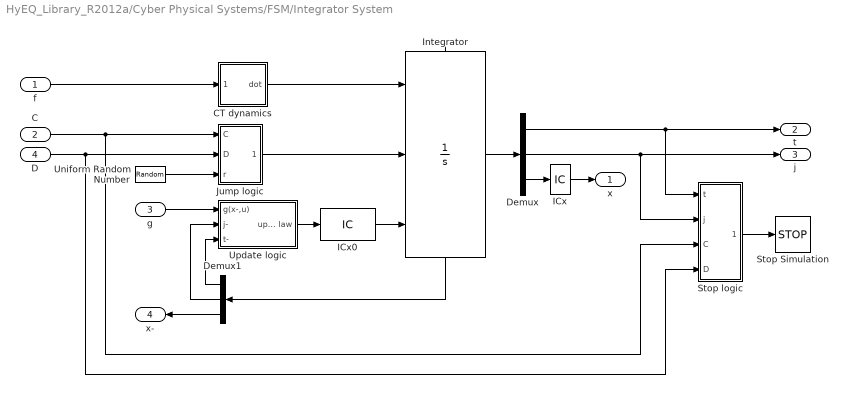
== system HyEQ_Library_R2012a/Cyber Physical Systems/FSM/Integrator System ==
  f : Inport
  C : Inport  Port=2
  g : Inport  Port=3
  D : Inport  Port=4
  CT dynamics : Subsystem
  Demux : Demux  Outputs=[1 1 -1]
  Demux1 : Demux  Outputs=[1 1 -1]
  ICx : InitialCondition  Value=x0
  ICx0 : InitialCondition  Value=[0; 0; x0(:)]
  Integrator : Integrator  ExternalReset=level hold  InitialConditionSource=external  ShowStatePort=on  ZeroCross=off
  Jump logic : Subsystem
  Stop Simulation : Stop
  Stop logic : Subsystem
  Uniform Random Number : UniformRandomNumber  Minimum=0  Seed=abs(floor(100*rand))  SampleTime=0
  Update logic : Subsystem
  x : Outport
  t : Outport  Port=2
  j : Outport  Port=3
  x- : Outport  Port=4
  wires:
  Demux1/2 -> Update logic/2(j-)
  Demux1/1 -> Update logic/3(t-)
  g/1 -> Update logic/1(g(x-,u))
  Uniform Random Number/1 -> Jump logic/3(r)
  Jump logic/1(jump) -> Integrator/2
  Demux1/3 -> x-/1
  f/1 -> CT dynamics/1(f(x,u))
  D/1 -> Jump logic/2(D), Stop logic/4(D)
  C/1 -> Jump logic/1(C), Stop logic/3(C)
  Integrator/1 -> Demux/1
  Stop logic/1(stop) -> Stop Simulation/1
  CT dynamics/1(dot) -> Integrator/1
  Update logic/1(update law) -> ICx0/1
  Demux/1 -> Stop logic/1(t), t/1
  Demux/2 -> Stop logic/2(j), j/1
  Integrator/State -> Demux1/1
  Demux/3 -> ICx/1
  ICx/1 -> x/1
  ICx0/1 -> Integrator/3

== system HyEQ_Library_R2012a/Cyber Physical Systems/FSM/Plot Solutions ==

== system HyEQ_Library_R2012a/Cyber Physical Systems/HSu/Initialize variables ==

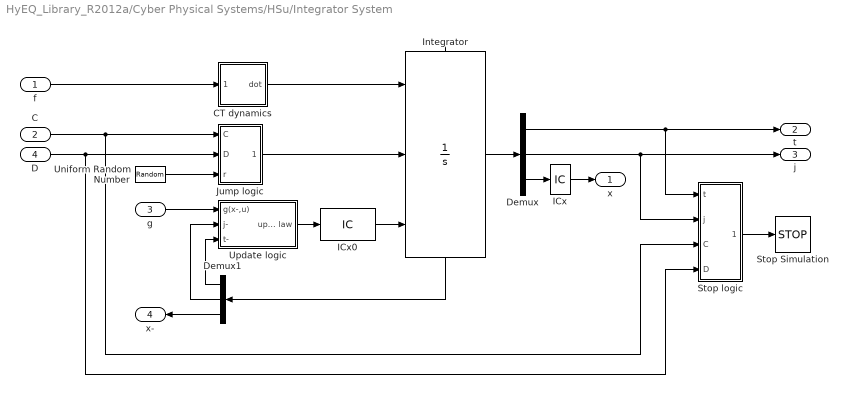
== system HyEQ_Library_R2012a/Cyber Physical Systems/HSu/Integrator System ==
  f : Inport
  C : Inport  Port=2
  g : Inport  Port=3
  D : Inport  Port=4
  CT dynamics : Subsystem
  Demux : Demux  Outputs=[1 1 -1]
  Demux1 : Demux  Outputs=[1 1 -1]
  ICx : InitialCondition  Value=x0
  ICx0 : InitialCondition  Value=[0; 0; x0(:)]
  Integrator : Integrator  ExternalReset=level hold  InitialConditionSource=external  ShowStatePort=on  ZeroCross=off
  Jump logic : Subsystem
  Stop Simulation : Stop
  Stop logic : Subsystem
  Uniform Random Number : UniformRandomNumber  Minimum=0  Seed=abs(floor(100*rand))  SampleTime=0
  Update logic : Subsystem
  x : Outport
  t : Outport  Port=2
  j : Outport  Port=3
  x- : Outport  Port=4
  wires:
  Demux1/2 -> Update logic/2(j-)
  Demux1/1 -> Update logic/3(t-)
  g/1 -> Update logic/1(g(x-,u))
  Uniform Random Number/1 -> Jump logic/3(r)
  Jump logic/1(jump) -> Integrator/2
  Demux1/3 -> x-/1
  f/1 -> CT dynamics/1(f(x,u))
  D/1 -> Jump logic/2(D), Stop logic/4(D)
  C/1 -> Jump logic/1(C), Stop logic/3(C)
  Integrator/1 -> Demux/1
  Stop logic/1(stop) -> Stop Simulation/1
  CT dynamics/1(dot) -> Integrator/1
  Update logic/1(update law) -> ICx0/1
  Demux/1 -> Stop logic/1(t), t/1
  Demux/2 -> Stop logic/2(j), j/1
  Integrator/State -> Demux1/1
  Demux/3 -> ICx/1
  ICx/1 -> x/1
  ICx0/1 -> Integrator/3

== system HyEQ_Library_R2012a/Cyber Physical Systems/HSu/Plot Solutions ==

== system HyEQ_Library_R2012a/Cyber Physical Systems/ZOH/Initialize variables ==
